simulink library "ltt"  (Simulink 8.1)
settings: Solver=ode1  StartTime=0.0  StopTime=Inf  FixedStep=0.001  RelTol=1e-3
PostLoadFcn:
  | , if any(exist('dsrtsu_mdlpostloadfcn', 'file') == [2, 3, 6]), try dsrtsu_mdlpostloadfcn('Execute', bdroot); catch fprintf('Error in PostLoadFcn (dsrtsu_mdlpostloadfcn) for model "%s":\n %s\n', bdroot, lasterr); end, end,
undefined symbols (not defined in the file or in its folder): C_TICK_TIME_S, FALSE, KACC_ACCTorqueMaintainTimer_ms, TRUE
libraries: simulink x1, hcu_lib x1
settings Model: DSRTSU_INTERNAL_RTI_VER=450  DSRTSU_INTERNAL_RTI_TYPE=rti1401  RTICANMMDATA=struct('GeneralSetupData',struct('modelroot','D:\ELN150201_TAIWAN\trunk\AdasDragon\software\sw_development\arch\app\acc','generalsettings',struct('filesettings',struct('destfolder',struct('Name','RTICANMM_FILES','Check',1),'buildfolder',struct('Name','.','Check',1),'AbsDestfolder',struct('Name','D:\ELN150201_TAIWAN\trunk\AdasDragon\software\sw_development\arch\app\acc\RTICANMM_FILES'),'AbsBuildfolder',struct('Name','D:\ELN150201_TAIWAN\trunk\AdasDragon\software\sw_development\arch\app\acc'))),'options',struct('addpaths',1,'rmpaths',1,'addtrcexclusion',logical(1),'cannavigator',struct('checkmonitoring',0),'show_usrtrc',0,'use_usrtrc',0),'advanced',struct('options',[1 1 1 1 1 1 1 1 1 1 1 1 1 1 1 1 1 1 1 1 1 1 1 1 1 1 1 1 1 1 1 1 1 1 1 1 1 1 1 1 1 1 1 1 1 1 1 1 1 1 1 1 1 1 1 1 1 1 1 1 1 1 1 1 1 1 1 1 1 1 1 1 1 1 1 1 1 1 1 1 1 1 1 1 1 1 1 1 1 1 1 1 1 1 1 1 1 1 1 1]),'MPSetup',{{}},'modelname','ltt','block','ltt'))  DSRTSU_INTERNAL_RTIFPGA=40  Creator=AT015555  LastModifiedBy=AT015555

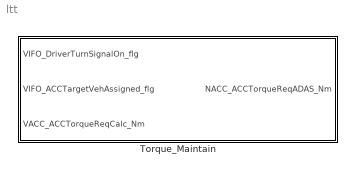
== system ltt ==
  Torque_Maintain : Subsystem

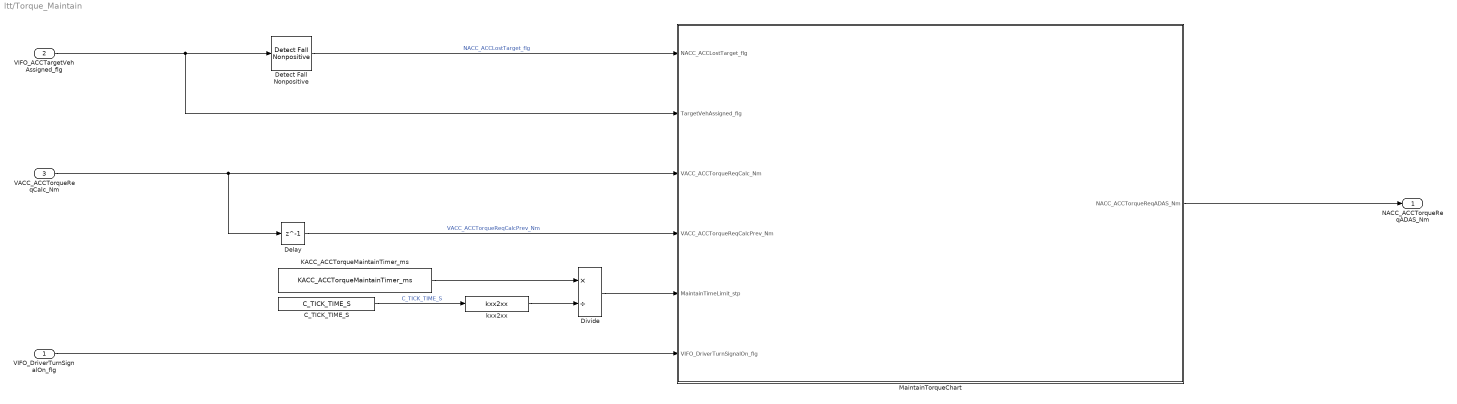
== system ltt/Torque_Maintain ==
  VIFO_DriverTurnSignalOn_flg : Inport
  VIFO_ACCTargetVehAssigned_flg : Inport  Port=2
  VACC_ACCTorqueReqCalc_Nm : Inport  Port=3
  C_TICK_TIME_S : Constant  Value=C_TICK_TIME_S
  Delay : Delay  DelayLength=1  InitialCondition=0
  Detect Fall Nonpositive : simulink/Logic and Bit Operations/Detect Fall Nonpositive  vinit=0  InputProcessing=Inherited  OutDataTypeStr=boolean
  Divide : Product  Inputs=*/
  KACC_ACCTorqueMaintainTimer_ms : Constant  Value=KACC_ACCTorqueMaintainTimer_ms
  MaintainTorqueChart : Stateflow chart  TreatAsAtomicUnit=on
  kxx2xx : hcu_lib/kxx2xx
  NACC_ACCTorqueReqADAS_Nm : Outport
  wires:
  Detect Fall Nonpositive/1 -> MaintainTorqueChart/1(NACC_ACCLostTarget_flg)  "NACC_ACCLostTarget_flg"
  MaintainTorqueChart/1(NACC_ACCTorqueReqADAS_Nm) -> NACC_ACCTorqueReqADAS_Nm/1
  VACC_ACCTorqueReqCalc_Nm/1 -> Delay/1, MaintainTorqueChart/3(VACC_ACCTorqueReqCalc_Nm)
  KACC_ACCTorqueMaintainTimer_ms/1 -> Divide/1
  kxx2xx/1 -> Divide/2
  Divide/1 -> MaintainTorqueChart/5(MaintainTimeLimit_stp)
  C_TICK_TIME_S/1 -> kxx2xx/1  "C_TICK_TIME_S"
  VIFO_ACCTargetVehAssigned_flg/1 -> Detect Fall Nonpositive/1, MaintainTorqueChart/2(TargetVehAssigned_flg)
  Delay/1 -> MaintainTorqueChart/4(VACC_ACCTorqueReqCalcPrev_Nm)  "VACC_ACCTorqueReqCalcPrev_Nm"
  VIFO_DriverTurnSignalOn_flg/1 -> MaintainTorqueChart/6(VIFO_DriverTurnSignalOn_flg)

== stateflow chart Torque_Maintain/MaintainTorqueChart ==
  state DIRECT_TORQUE
    du:
    NACC_ACCTorqueReqADAS_Nm = VACC_ACCTorqueReqCalc_Nm;
  state MAINTAIN_LAST_VALUE
    en:
    MaintainTimeLocal_stp = 0;
    du:
    MaintainTimeLocal_stp=MaintainTimeLocal_stp+1;
    ex:
    NACC_ACCTorqueReqADAS_Nm = VACC_ACCTorqueReqCalc_Nm;
  state GET_LAST_VALUE
    en:
    NACC_ACCTorqueReqADAS_Nm = VACC_ACCTorqueReqCalcPrev_Nm;
  (default) -> DIRECT_TORQUE
  (junction 16) -> DIRECT_TORQUE : [MaintainTimeLocal_stp>MaintainTimeLimit_stp...
      | ||TargetVehAssigned_flg==TRUE]
  MAINTAIN_LAST_VALUE -> (junction 16)
  DIRECT_TORQUE -> (junction 17)
  (junction 17) -> GET_LAST_VALUE : [NACC_ACCLostTarget_flg==TRUE ...
      | && VIFO_DriverTurnSignalOn_flg == FALSE]
  GET_LAST_VALUE -> MAINTAIN_LAST_VALUE
  data: NACC_ACCTorqueReqADAS_Nm output single; NACC_ACCLostTarget_flg input boolean; TargetVehAssigned_flg input boolean; VACC_ACCTorqueReqCalc_Nm input single; VACC_ACCTorqueReqCalcPrev_Nm input double; FALSE parameter double; TRUE parameter double; MaintainTimeLocal_stp local single; MaintainTimeLimit_stp input single; VIFO_DriverTurnSignalOn_flg input double
